simulink model "BLDC_abc_dq_comparison_vB"  (R2021a)
settings: Solver=FixedStepAuto  StartTime=0.0  StopTime=15  FixedStep=0.00001  RelTol=1e-3
settings Model: Creator=raca  LastModifiedBy=headl
settings SolverCC: AlgebraicLoopSolver=TrustRegion
settings DataIOCC: ReturnWorkspaceOutputs=off
settings DebuggingCC: SFMachineParentedDataDiag=warning  ArithmeticOperatorsInVariantConditions=warning
settings SFSimCC: SimUseLocalCustomCode=off  CustomCodeUndefinedFunction=UseInterfaceOnly
settings RTWCC: RTWUseLocalCustomCode=off
settings CodeAppCC: StateflowObjectComments=on

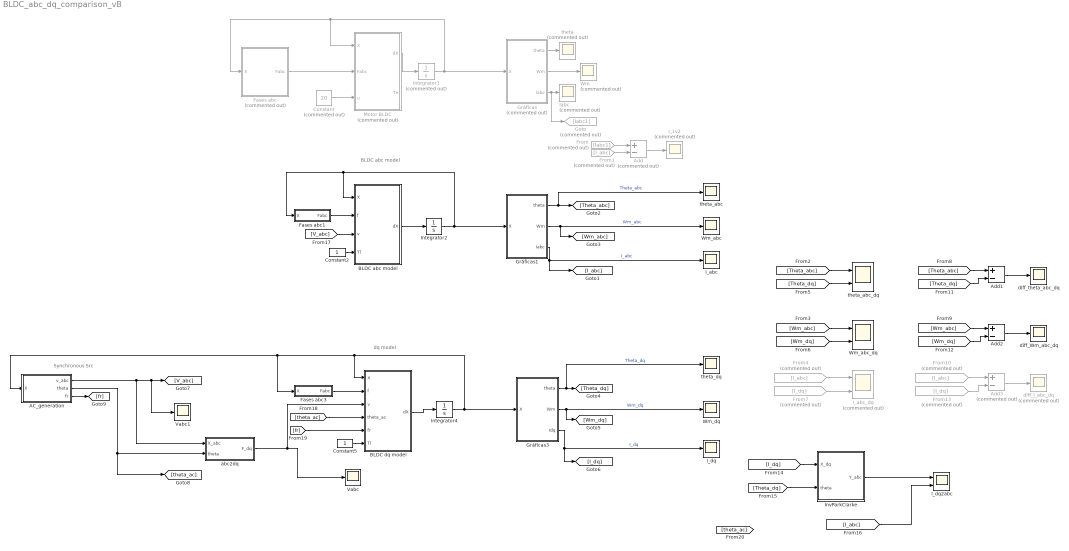
== system BLDC_abc_dq_comparison_vB ==
  note: BLDC abc model
  note: Synchronous Src
  note: dq model
  AC_generation : Subsystem  mask{isSync=on, fr=100}
      mask prompts: isSync "Synchronous"
  Add : Sum  Commented=on  Inputs=+-
  Add1 : Sum  Inputs=+-
  Add2 : Sum  Inputs=+-
  Add3 : Sum  Commented=on  Inputs=+-
  BLDC abc model : MATLAB Function  TreatAsAtomicUnit=on
  BLDC dq model : MATLAB Function  TreatAsAtomicUnit=on
  Constant : Constant  Commented=on  Value=20
  Constant2 : Constant
  Constant5 : Constant
  Fases abc : MATLAB Function  Commented=on  TreatAsAtomicUnit=on
  Fases abc1 : MATLAB Function  TreatAsAtomicUnit=on
  Fases abc3 : MATLAB Function  TreatAsAtomicUnit=on
  From : From  Commented=on  GotoTag=Iabc1
  From1 : From  Commented=on  GotoTag=I_abc
  From10 : From  Commented=on  GotoTag=I_abc
  From13 : From  Commented=on  GotoTag=I_dq
  From4 : From  Commented=on  GotoTag=I_abc
  From7 : From  Commented=on  GotoTag=I_dq
  Goto : Goto  Commented=on  GotoTag=Iabc1
  Gráficas : MATLAB Function  Commented=on  TreatAsAtomicUnit=on
  Gráficas1 : MATLAB Function  TreatAsAtomicUnit=on
  Gráficas3 : MATLAB Function  TreatAsAtomicUnit=on
  I_1v2 : Scope  Commented=on
  I_abc : Scope
  I_abc_dq : Scope  Commented=on  NumInputPorts=2
  I_dq : Scope
  I_dq2abc : Scope  NumInputPorts=2
  Iabc : Scope  Commented=on
  Integrator1 : Integrator  Commented=on  InitialCondition=[0 0.1 0 0 0]
  Integrator2 : Integrator  InitialCondition=[0;0;0;0.1;0]
  Integrator4 : Integrator  InitialCondition=[0;0;0.1;0]
  InvParkClarke : MATLAB Function  TreatAsAtomicUnit=on
  Motor BLDC : MATLAB Function  Commented=on  TreatAsAtomicUnit=on
  Vabc : Scope
  Vabc1 : Scope
  Wm : Scope  Commented=on
  Wm_abc : Scope
  Wm_abc_dq : Scope  NumInputPorts=2
  Wm_dq : Scope
  abc2dq : MATLAB Function  TreatAsAtomicUnit=on
  diff_I_abc_dq : Scope  Commented=on
  diff_Wm_abc_dq : Scope
  diff_theta_abc_dq : Scope
  theta : Scope  Commented=on
  theta_abc : Scope
  theta_abc_dq : Scope  NumInputPorts=2
  theta_dq : Scope
  wires:
  Fases abc/1(Fabc) -> Motor BLDC/2(Fabc)
  Motor BLDC/1(dX) -> Integrator1/1
  Integrator1/1 -> Motor BLDC/1(X), Fases abc/1(X), Gráficas/1(X)
  Gráficas/1(theta) -> theta/1
  Gráficas/2(Wm) -> Wm/1
  Gráficas/3(Iabc) -> Goto/1, Iabc/1
  Constant/1 -> Motor BLDC/3(u)
  BLDC abc model/1(dX) -> Integrator2/1
  Fases abc1/1(Fabc) -> BLDC abc model/2(f)
  Gráficas1/2(Wm) -> [Wm_abc], Wm_abc/1  "Wm_abc"
  Integrator2/1 -> BLDC abc model/1(X), Fases abc1/1(X), Gráficas1/1(X)
  Gráficas1/1(theta) -> theta_abc/1, [Theta_abc]  "Theta_abc"
  Constant2/1 -> BLDC abc model/4(Tl)
  Gráficas1/3(Iabc) -> [I_abc], I_abc/1  "I_abc"
  Gráficas3/1(theta) -> [Theta_dq], theta_dq/1  "Theta_dq"
  Constant5/1 -> BLDC dq model/6(Tl)
  BLDC dq model/1(dX) -> Integrator4/1
  Integrator4/1 -> BLDC dq model/1(X), AC_generation/1(X), Fases abc3/1(X), Gráficas3/1(X)
  Gráficas3/3(Idq) -> [I_dq], I_dq/1  "I_dq"
  Gráficas3/2(Wm) -> Wm_dq/1, [Wm_dq]  "Wm_dq"
  From/1 -> Add/1
  From1/1 -> Add/2
  Add/1 -> I_1v2/1
  [Theta_abc] -> theta_abc_dq/1
  [Theta_dq] -> theta_abc_dq/2
  [Wm_abc] -> Wm_abc_dq/1
  [Wm_dq] -> Wm_abc_dq/2
  From4/1 -> I_abc_dq/1
  From7/1 -> I_abc_dq/2
  [Theta_abc] -> Add1/1
  [Theta_dq] -> Add1/2
  [Wm_abc] -> Add2/1
  [Wm_dq] -> Add2/2
  From10/1 -> Add3/1
  From13/1 -> Add3/2
  Add1/1 -> diff_theta_abc_dq/1
  Add2/1 -> diff_Wm_abc_dq/1
  Add3/1 -> diff_I_abc_dq/1
  [I_dq] -> InvParkClarke/1(X_dq)
  InvParkClarke/1(Y_abc) -> I_dq2abc/1
  [I_abc] -> I_dq2abc/2
  Fases abc3/1(Fabc) -> BLDC dq model/2(f)
  AC_generation/1(v_abc) -> abc2dq/1(X_abc), Vabc1/1, [V_abc]
  abc2dq/1(F_dq) -> Vabc/1, BLDC dq model/3(v)
  AC_generation/2(theta) -> [theta_ac], abc2dq/2(theta)
  [V_abc] -> BLDC abc model/3(v)
  [theta_ac] -> BLDC dq model/4(theta_ac)
  [Theta_dq] -> InvParkClarke/2(theta)
  AC_generation/3(fr) -> [fr]
  [fr] -> BLDC dq model/5(fr)

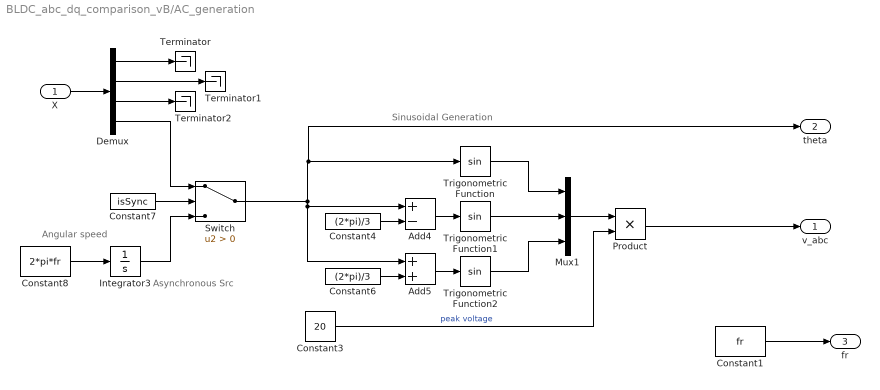
== system BLDC_abc_dq_comparison_vB/AC_generation ==
  note: Sinusoidal Generation
  note: Angular speed
  note: Asynchronous Src
  X : Inport
  Add4 : Sum  Inputs=+-
  Add5 : Sum
  Constant1 : Constant  Value=fr
  Constant3 : Constant  Value=20
  Constant4 : Constant  Value=(2*pi)/3
  Constant6 : Constant  Value=(2*pi)/3
  Constant7 : Constant  Value=isSync
  Constant8 : Constant  Value=2*pi*fr
  Demux : Demux
  Integrator3 : Integrator
  Mux1 : Mux  Inputs=3
  Product : Product
  Switch : Switch  Criteria=u2 > Threshold
  Terminator : Terminator
  Terminator1 : Terminator
  Terminator2 : Terminator
  Trigonometric Function : Trigonometry
  Trigonometric Function1 : Trigonometry
  Trigonometric Function2 : Trigonometry
  v_abc : Outport
  theta : Outport  Port=2
  fr : Outport  Port=3
  wires:
  Constant8/1 -> Integrator3/1
  Switch/1 -> Add5/1, Add4/1, theta/1, Trigonometric Function/1
  Constant3/1 -> Product/2  "peak voltage"
  Integrator3/1 -> Switch/3
  Demux/4 -> Switch/1
  Add5/1 -> Trigonometric Function2/1
  Trigonometric Function/1 -> Mux1/1
  Mux1/1 -> Product/1
  Trigonometric Function1/1 -> Mux1/2
  Trigonometric Function2/1 -> Mux1/3
  Constant7/1 -> Switch/2
  X/1 -> Demux/1
  Constant4/1 -> Add4/2
  Add4/1 -> Trigonometric Function1/1
  Constant6/1 -> Add5/2
  Product/1 -> v_abc/1
  Demux/1 -> Terminator/1
  Demux/3 -> Terminator2/1
  Demux/2 -> Terminator1/1
  Constant1/1 -> fr/1

== matlab function BLDC_abc_dq_comparison_vB/Fases abc3 ==
  data: X input; Fabc output
function Fabc = fcn(X)
Fabc = [0;0;0];
    theta = mod(X(4),2*pi);
    %theta = mod(X,2*pi);
    
    if (0<=theta)&&(theta<(pi/6))
        Fa = (6/pi)*theta;
    elseif ((pi/6)<=theta)&&(theta<(5*pi/6))
        Fa = 1;
    elseif ((5*pi/6<=theta))&&(theta<(7*pi/6))
        Fa = (6/pi)*(pi-theta);
    elseif ((7*pi/6)<=theta)&&(theta<(11*pi/6))
        Fa = -1;
    elseif ((11*pi/6)<=theta)&&(theta<(2*pi))
        Fa = (6/pi)*(theta-2*pi);
    else
        Fa = NaN;
    end
    
    if (0<=theta)&&(theta<(3*pi/6))
        Fb = -1;
    elseif ((3*pi/6)<=theta)&&(theta<(5*pi/6))
        Fb = (6/pi)*(theta-(2*pi)/3);
    elseif ((5*pi/6)<=theta)&&(theta<(9*pi/6))
        Fb = 1;
    elseif ((9*pi/6)<=theta)&&(theta<(11*pi/6))
        Fb = (6/pi)*(-theta+(5*pi)/3);
    elseif ((11*pi/6)<=theta)&&(theta<(2*pi))
        Fb = -1;
    else
        Fb = NaN;
    end
    
    if (0<=theta)&&(theta<(pi/6))
        Fc = 1;
    elseif ((pi/6)<=theta)&&(theta<(3*pi/6))
        Fc = (6/pi)*(pi/3-theta);
    elseif ((3*pi/6)<=theta)&&(theta<(7*pi/6))
        Fc = -1;
    elseif ((7*pi/6)<=theta)&&(theta<(9*pi/6))
        Fc = (6/pi)*(theta-(4*pi)/3);
    elseif ((9*pi/6)<=theta)&&(theta<(2*pi))
        Fc = 1;
    else
        Fc = NaN; 
    end
    
    Fabc = [Fa;Fb;Fc];
end

== matlab function BLDC_abc_dq_comparison_vB/Gráficas3 ==
  data: X input; theta output; Wm output; Idq output
function [theta,Wm,Idq] = DEMUX(X)
theta = X(4); Wm = X(3);Idq = X(1:2);

== matlab function BLDC_abc_dq_comparison_vB/Motor BLDC ==
  data: X input; dX output; Fabc input; u input; Te output
function [dX,Te] = fcn(X,Fabc,u)
Wm = X(2);Iabc = X(3:5);
R = 0.7;
L = 0.00272-0.0015; %=L-Lm
J = 0.000284;
b = 0.02;
P = 4;
Lambda = 0.105;

Tl = 1; %No carga

Vabc = u*Fabc;

Eabc = Lambda*Wm*Fabc;
dTheta = P*Wm/2;
Te = (Iabc'*Eabc)/Wm;
dWm = (Te-b*Wm-Tl)/J;
dIabc = (-R*Iabc - Eabc + Vabc)/L;

dX = [dTheta;dWm;dIabc];
end

== matlab function BLDC_abc_dq_comparison_vB/Gráficas ==
  data: X input; theta output; Wm output; Iabc output
function [theta,Wm,Iabc] = DEMUX(X)
theta = X(1); Wm = X(2);Iabc = X(3:5);

== matlab function BLDC_abc_dq_comparison_vB/Fases abc ==
  data: X input; Fabc output
function Fabc = fcn(X)
    theta = mod(X(1),2*pi);
    
    if (0<=theta)&&(theta<(pi/6))
        Fa = (6/pi)*theta;
    elseif ((pi/6)<=theta)&&(theta<(5*pi/6))
        Fa = 1;
    elseif ((5*pi/6<=theta))&&(theta<(7*pi/6))
        Fa = (6/pi)*(pi-theta);
    elseif ((7*pi/6)<=theta)&&(theta<(11*pi/6))
        Fa = -1;
    elseif ((11*pi/6)<=theta)&&(theta<(2*pi))
        Fa = (6/pi)*(theta-2*pi);
    else
        Fa = NaN;
    end
    
    if (0<=theta)&&(theta<(3*pi/6))
        Fb = -1;
    elseif ((3*pi/6)<=theta)&&(theta<(5*pi/6))
        Fb = (6/pi)*(theta-(2*pi)/3);
    elseif ((5*pi/6)<=theta)&&(theta<(9*pi/6))
        Fb = 1;
    elseif ((9*pi/6)<=theta)&&(theta<(11*pi/6))
        Fb = (6/pi)*(-theta+(5*pi)/3);
    elseif ((11*pi/6)<=theta)&&(theta<(2*pi))
        Fb = -1;
    else
        Fb = NaN;
    end
    
    if (0<=theta)&&(theta<(pi/6))
        Fc = 1;
    elseif ((pi/6)<=theta)&&(theta<(3*pi/6))
        Fc = (6/pi)*(pi/3-theta);
    elseif ((3*pi/6)<=theta)&&(theta<(7*pi/6))
        Fc = -1;
    elseif ((7*pi/6)<=theta)&&(theta<(9*pi/6))
        Fc = (6/pi)*(theta-(4*pi)/3);
    elseif ((9*pi/6)<=theta)&&(theta<(2*pi))
        Fc = 1;
    else
        Fc = NaN; 
    end
    
    Fabc = [Fa;Fb;Fc];
end

== matlab function BLDC_abc_dq_comparison_vB/BLDC abc model ==
  data: X input; f input; v input; dX output; Tl input
function dX = fcn(X,f,v,Tl)
u = [v;Tl]; 
i_a = X(1); i_b = X(2); i_c = X(3); wm = X(4); theta = X(5);

lamda = 0.105;
R = 0.7;
L = 0.00272;
M = 0.0015;
J = 0.000284;
P = 4;
b = 0.02;

%e = [(lamda*wm).*f;0;0];

A =[-(R/(L-M)) 0 0 -(lamda/(L-M))*f(1) 0;...
    0 -(R/(L-M)) 0 -(lamda/(L-M))*f(2) 0;...
    0 0 -(R/(L-M)) -(lamda/(L-M))*f(3) 0;...
    (lamda/J)*f(1) (lamda/J)*f(2) (lamda/J)*f(3) -b/J 0;...
    0 0 0 P/2 0];

B = diag([1/(L-M) 1/(L-M) 1/(L-M) -1/J]);
B = [B;0 0 0 0];


dX = [0;0;0;0;0];
dX = A*X + B*u;

end

== matlab function BLDC_abc_dq_comparison_vB/Fases abc1 ==
  data: X input; Fabc output
function Fabc = fcn(X)
Fabc = [0;0;0];
    theta = mod(X(5),2*pi);
    
    if (0<=theta)&&(theta<(pi/6))
        Fa = (6/pi)*theta;
    elseif ((pi/6)<=theta)&&(theta<(5*pi/6))
        Fa = 1;
    elseif ((5*pi/6<=theta))&&(theta<(7*pi/6))
        Fa = (6/pi)*(pi-theta);
    elseif ((7*pi/6)<=theta)&&(theta<(11*pi/6))
        Fa = -1;
    elseif ((11*pi/6)<=theta)&&(theta<(2*pi))
        Fa = (6/pi)*(theta-2*pi);
    else
        Fa = NaN;
    end
    
    if (0<=theta)&&(theta<(3*pi/6))
        Fb = -1;
    elseif ((3*pi/6)<=theta)&&(theta<(5*pi/6))
        Fb = (6/pi)*(theta-(2*pi)/3);
    elseif ((5*pi/6)<=theta)&&(theta<(9*pi/6))
        Fb = 1;
    elseif ((9*pi/6)<=theta)&&(theta<(11*pi/6))
        Fb = (6/pi)*(-theta+(5*pi)/3);
    elseif ((11*pi/6)<=theta)&&(theta<(2*pi))
        Fb = -1;
    else
        Fb = NaN;
    end
    
    if (0<=theta)&&(theta<(pi/6))
        Fc = 1;
    elseif ((pi/6)<=theta)&&(theta<(3*pi/6))
        Fc = (6/pi)*(pi/3-theta);
    elseif ((3*pi/6)<=theta)&&(theta<(7*pi/6))
        Fc = -1;
    elseif ((7*pi/6)<=theta)&&(theta<(9*pi/6))
        Fc = (6/pi)*(theta-(4*pi)/3);
    elseif ((9*pi/6)<=theta)&&(theta<(2*pi))
        Fc = 1;
    else
        Fc = NaN; 
    end
    
    Fabc = [Fa;Fb;Fc];
end

== matlab function BLDC_abc_dq_comparison_vB/Gráficas1 ==
  data: X input; theta output; Wm output; Iabc output
function [theta,Wm,Iabc] = DEMUX(X)
theta = X(5); Wm = X(4);Iabc = X(1:3);

== matlab function BLDC_abc_dq_comparison_vB/InvParkClarke ==
  data: X_dq input; Y_abc output; theta input
function Y_abc = fcn(X_dq, theta)
X_dq0 = [X_dq;0];

iT_PC = sqrt(2/3)*[cos(theta)          -sin(theta)            1/sqrt(2); ...
                  cos(theta-2*pi/3)   -sin(theta-2*pi/3)     1/sqrt(2); ...
                  cos(theta+2*pi/3)   -sin(theta+2*pi/3)     1/sqrt(2)];


Y_abc =iT_PC*X_dq0;
end

== matlab function BLDC_abc_dq_comparison_vB/abc2dq ==
  data: X_abc input; F_dq output; theta input
function F_dq = fcn(X_abc, theta)

% Park clarke transform eliminating the third element
PC_T = (sqrt(2)/2)*[sqrt(3)*cos(theta)  sin(theta)  -sin(theta) ; ...
                    -sqrt(3)*sin(theta)  cos(theta)  -cos(theta)];

F_dq = PC_T*X_abc;
                
end

== matlab function BLDC_abc_dq_comparison_vB/BLDC dq model ==
  data: X input; f input; v input; theta_ac input; fr input; dX output; Tl input
function dX = fcn(X,f,v,theta_ac,fr,Tl)
i_d = X(1); i_q = X(2); wm = X(3); theta = X(4);
i_dq = X(1:2);

lamda = 0.105;
R = 0.7;
L = 0.00272;
M = 0.0015;
J = 0.000284;
P = 4;
b = 0.02;


M_LR = [-R/(L-M)  (2*pi*fr); -(2*pi*fr)  -R/(L-M)];

% Park clarke transform eliminating the third element
PC_T = (sqrt(2)/2)*[sqrt(3)*cos(theta_ac)  sin(theta_ac)  -sin(theta_ac) ; ...
                    -sqrt(3)*sin(theta_ac)  cos(theta_ac)  -cos(theta_ac)];
                
                
                % Park clarke transform eliminating the third element
PC_Te = (sqrt(2)/2)*[sqrt(3)*cos(theta)  sin(theta)  -sin(theta) ; ...
                    -sqrt(3)*sin(theta)  cos(theta)  -cos(theta)];


e_dq =(lamda*wm)*PC_Te*f;
% v_dq = v*(PC_T*f);
v_dq = v;

di_dq = M_LR*i_dq + (1/(L-M))*v_dq - (1/(L-M))*e_dq;
T_e = (e_dq'*i_dq)/wm;
dwm = (T_e - Tl -b*wm)/J;
dtheta = (P/2)*wm;

dX = [di_dq;dwm;dtheta];

end
